simulink model "Rail_Sim"  (R2024a)
settings: Solver=VariableStepAuto  StartTime=0.0  StopTime=50  MaxStep=0.01  RelTol=1e-9
model workspace (MAT data in the model file):
  Cd = 0.6
  S = 0.00817128249199
  T_data = [20.408; 7112.245; 6734.694; 6897.959; 6612.245; 6765.306; 6540.816; 6581.633; 6520.408; 6795.918; 7091.837; 7285.714; 7408.163; 7581.633; 7622.449; 7724.49; 7653.061; 7540.816; 7500; 7336.735; 7224.49; 6785.714; 6326.531; 5897.959; 5704.082; 3540.816; 3408.163; 2887.755; 2234.694; 1673.469; 1489.796; 1418.367; 1295.918; 816.327; 653.061; 581.633; 489.796; 285.714; 20.408; 0]
  T_time = [0.009; 0.044; 0.063; 0.078; 0.094; 0.109; 0.125; 0.147; 0.194; 0.35; 0.428; 0.563; 0.694; 0.988; 1.266; 1.491; 1.581; 1.641; 1.684; 1.716; 1.784; 1.938; 2.138; 2.491; 2.6; 2.919; 3.022; 3.138; 3.3; 3.388; 3.441; 3.544; 3.609; 3.688; 3.778; 3.819; 3.853; 3.897; 3.981; 3.997]
  e = 1.55334303427
  l = 6.096
  m_data = [23.6873 23.687272 23.682428 23.675988 23.669548 23.663108 23.656696 23.650256 23.643816 23.637376 23.630936 23.61842 ... (250 elements, 250x1)]
  m_time = [0.004; 0.008; 0.012; 0.016; 0.02; 0.024; 0.028; 0.032; 0.036; 0.04; 0.044; 0.048; 0.052; 0.056; 0.06; 0.064; 0.068; 0.072; 0.076; 0.08; 0.084; 0.088; 0.092; 0.096; 0.1; 0.104; 0.108; 0.112; 0.116; 0.12; 0.124; 0.128; 0.132; 0.136; 0.14; 0.144; 0.148; 0.152; 0.156; 0.16; 0.164; 0.168; 0.172; 0.176; 0.18; 0.184; 0.188; 0.192; 0.196; 0.2; 0.204; 0.208; 0.212; 0.216; 0.22; 0.224; 0.228; 0.232; 0.236; 0.24; 0.246; 0.255; 0.269; 0.289; 0.309; 0.329; 0.349; 0.369; 0.389; 0.409; 0.429; 0.449; 0.469; 0.489; 0.509; 0.529; 0.549; 0.569; 0.589; 0.609; 0.629; 0.649; 0.669; 0.689; 0.709; 0.729; 0.749; 0.769; 0.789; 0.809; 0.829; 0.849; 0.869; 0.889; 0.909; 0.929; 0.949; 0.969; 0.989; 1.009; 1.029; 1.049; 1.069; 1.089; 1.109; 1.129; 1.149; 1.169; 1.189; 1.209; 1.228; 1.247; 1.267; 1.287; 1.307; 1.327; 1.347; 1.364; 1.38; 1.397; 1.417; 1.437; 1.457; 1.477; 1.495; 1.513; 1.533; 1.553; 1.573; 1.593; 1.612; 1.631; 1.651; 1.671; 1.691; 1.711; 1.731; 1.751; 1.771; 1.791; 1.811; 1.831; 1.851; 1.871; 1.891; 1.911; 1.931; 1.951; 1.971; 1.991; 2.011; 2.031; 2.051; 2.071; 2.091; 2.111; 2.131; 2.151; 2.171; 2.191; 2.211; 2.231; 2.251; 2.271; 2.291; 2.311; 2.331; 2.351; 2.371; 2.391; 2.411; 2.431; 2.451; 2.471; 2.491; 2.511; 2.531; 2.551; 2.571; 2.591; 2.611; 2.631; 2.651; 2.671; 2.691; 2.711; 2.731; 2.751; 2.771; 2.791; 2.811; 2.831; 2.851; 2.871; 2.891; 2.911; 2.931; 2.951; 2.971; 2.991; 3.011; 3.031; 3.051; 3.071; 3.091; 3.111; 3.131; 3.151; 3.171; 3.191; 3.211; 3.231; 3.251; 3.271; 3.291; 3.311; 3.331; 3.351; 3.371; 3.391; 3.411; 3.431; 3.451; 3.471; 3.491; 3.511; 3.531; 3.551; 3.571; 3.591; 3.611; 3.631; 3.651; 3.671; 3.691; 3.711; 3.731; 3.751; 3.771; 3.791; 3.811; 3.831; 3.851; 3.871; 3.891; 3.911; 3.931; 3.951; 3.971; 3.991]
  mu = 0.4
libraries: simulink x1
settings Model: Creator=thatf  LastModifiedBy=thatf
settings ModelReferenceCC: EnableRefExpFcnMdlSchedulingChecks=on
settings RTWCC: GPUComputeCapability=3.5

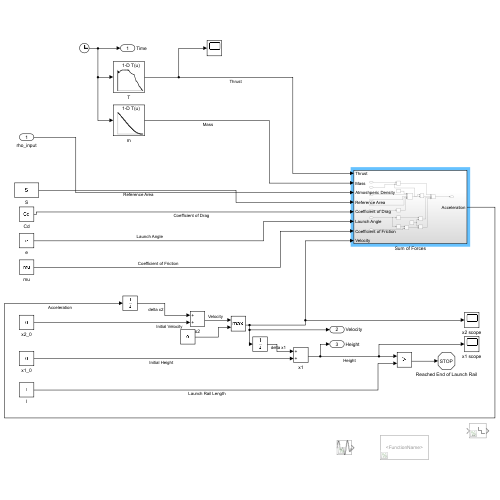
[thumbnail: Simulink's stored preview of the top-level diagram]
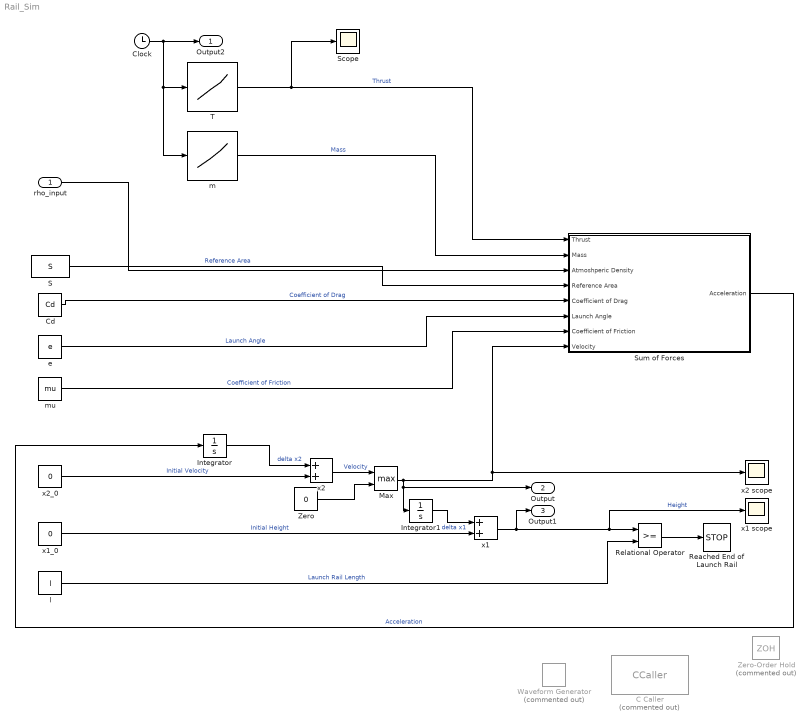
== system Rail_Sim ==
  rho_input : Inport
  C Caller : CCaller  Commented=on
  Cd : Constant  Value=Cd
  Clock : Clock
  Integrator : Integrator
  Integrator1 : Integrator
  Max : MinMax  Function=max  Inputs=2
  Reached End of Launch Rail : Stop
  Relational Operator : RelationalOperator  OutDataTypeStr=boolean  RndMeth=Simplest  InputSameDT=off
  S : Constant  Value=S
  Scope : Scope
  Sum of Forces : Subsystem
  T : Lookup_n-D  NumberOfTableDimensions=1  BreakpointsForDimension1=T_time  Table=T_data  InternalRulePriority=Speed  RndMeth=Simplest
  Waveform Generator : simulink/Sources/Waveform Generator  Commented=on  OutMin=[]  OutMax=[]  OutDataTypeStr=double  SelectedSignal=1  BlockNames=MultiportSwitch_e3df3653d217406  SampleTime=0.1
  Zero : Constant  Value=0  OutDataTypeStr=Inherit: Inherit via back propagation
  Zero-Order Hold : ZeroOrderHold  Commented=on  SampleTime=-1
  e : Constant  Value=e
  l : Constant  Value=l
  m : Lookup_n-D  NumberOfTableDimensions=1  BreakpointsForDimension1=m_time  Table=m_data  InternalRulePriority=Speed  RndMeth=Simplest
  mu : Constant  Value=mu
  x1 : Sum
  x1 scope : Scope
  x1_0 : Constant  Value=0
  x2 : Sum
  x2 scope : Scope
  x2_0 : Constant  Value=0
  Output2 : Outport  SignalName=Time
  Output : Outport  Port=2  SignalName=Velocity
  Output1 : Outport  Port=3  SignalName=Height
  wires:
  x2_0/1 -> x2/2  "Initial Velocity"
  x1_0/1 -> x1/2  "Initial Height"
  x1/1 -> Output1/1, Relational Operator/1, x1 scope/1  "Height"
  Integrator1/1 -> x1/1  "delta x1"
  Relational Operator/1 -> Reached End of Launch Rail/1
  l/1 -> Relational Operator/2  "Launch Rail Length"
  Clock/1 -> Output2/1, m/1, T/1
  T/1 -> Scope/1, Sum of Forces/1(Thrust)  "Thrust"
  m/1 -> Sum of Forces/2(Mass)  "Mass"
  S/1 -> Sum of Forces/4(Reference Area)  "Reference Area"
  Cd/1 -> Sum of Forces/5(Coefficient of Drag)  "Coefficient of Drag"
  e/1 -> Sum of Forces/6(Launch Angle)  "Launch Angle"
  mu/1 -> Sum of Forces/7(Coefficient of Friction)  "Coefficient of Friction"
  Sum of Forces/1(" Acceleration") -> Integrator/1  "Acceleration"
  Integrator/1 -> x2/1  "delta x2"
  rho_input/1 -> Sum of Forces/3(Atmoshperic Density)
  Zero/1 -> Max/2
  x2/1 -> Max/1  "Velocity"
  Max/1 -> Sum of Forces/8(Velocity), x2 scope/1, Output/1, Integrator1/1

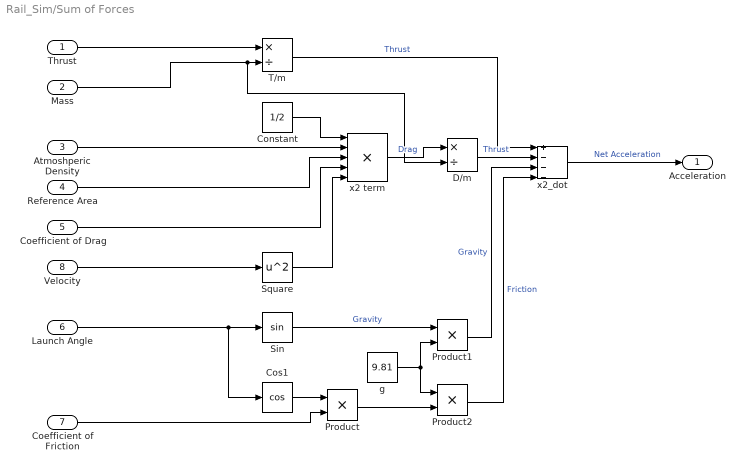
== system Rail_Sim/Sum of Forces ==
  Thrust : Inport
  Mass : Inport  Port=2
  Atmoshperic Density : Inport  Port=3
  Reference Area : Inport  Port=4
  Coefficient of Drag : Inport  Port=5
  Launch Angle : Inport  Port=6
  Coefficient of Friction : Inport  Port=7
  Velocity : Inport  Port=8
  Constant : Constant  Value=1/2
  Cos1 : Trigonometry  Operator=cos
  D/m : Product  Inputs=*/  RndMeth=Zero  SaturateOnIntegerOverflow=on
  Product : Product
  Product1 : Product
  Product2 : Product
  Sin : Trigonometry
  Square : Math  Operator=square
  T/m : Product  Inputs=*/  RndMeth=Zero  SaturateOnIntegerOverflow=on
  g : Constant  Value=9.81
  x2 term : Product  Inputs=5
  x2_dot : Sum  Inputs=+---
  " Acceleration" : Outport
  wires:
  Coefficient of Friction/1 -> Product/2
  Sin/1 -> Product1/1  "Gravity"
  Square/1 -> x2 term/5
  Coefficient of Drag/1 -> x2 term/4
  x2 term/1 -> D/m/1  "Drag"
  T/m/1 -> x2_dot/1  "Thrust"
  Atmoshperic Density/1 -> x2 term/2
  Velocity/1 -> Square/1
  Launch Angle/1 -> Cos1/1, Sin/1
  Mass/1 -> D/m/2, T/m/2
  Product/1 -> Product2/2
  Cos1/1 -> Product/1
  Reference Area/1 -> x2 term/3
  Thrust/1 -> T/m/1
  x2_dot/1 -> " Acceleration"/1  "Net Acceleration"
  g/1 -> Product1/2, Product2/1
  Product1/1 -> x2_dot/3  "Gravity"
  Product2/1 -> x2_dot/4  "Friction"
  Constant/1 -> x2 term/1
  D/m/1 -> x2_dot/2  "Thrust"
